simulink model "sldemo_variant_subsystems"  (Simulink 7.6)
settings: Solver=FixedStepDiscrete  StartTime=0.0  StopTime=10.0  RelTol=1e-3
PreLoadFcn:
  | VSS_NONLINEAR_CONTROLLER=Simulink.Variant('VSS_MODE==1')
  | VSS_SECOND_ORDER_CONTROLLER=Simulink.Variant('VSS_MODE==2')
  | 
  | VSS_MODE=1
Description:
  | Variant Subsystems
  | 
  | This demo illustrates Simulink(R) variant subsystems. Variant subsystems let
  | you provide multiple implementations to a subsystem where only one
  | implementation is active during simulation. You can programmatically swap out
  | the active implementation and replace it with one of the other implementations
  | without modifying the model.
settings Model: Creator=The MathWorks Inc.
settings OptimizationCC: InlineParams=on
settings RTWCC: ProcessScript=grt_make_rtw_hook

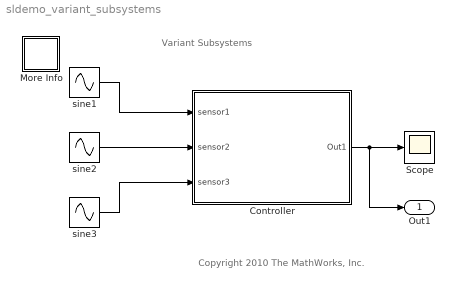
== system sldemo_variant_subsystems ==
  note: Copyright 2010 The MathWorks, Inc.
  note: Variant Subsystems
  Controller : Subsystem  Variant=on
  More Info : Subsystem
      settings: OpenFcn=showdemo(bdroot(gcb))
      mask Display: disp('?')
  Scope : Scope
  sine1 : Sin  Amplitude=.1  Frequency=pi/3  SampleTime=.01
  sine2 : Sin  Amplitude=2  SampleTime=.01
  sine3 : Sin  Amplitude=.3  Frequency=pi/6  SampleTime=.01
  Out1 : Outport
  wires:
  sine2/1 -> Controller/2(sensor2)
  sine1/1 -> Controller/1(sensor1)
  sine3/1 -> Controller/3(sensor3)
  Controller/1(Out1) -> Scope/1, Out1/1

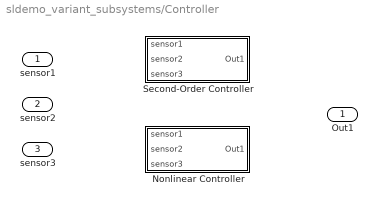
== system sldemo_variant_subsystems/Controller ==
  sensor1 : Inport
  sensor2 : Inport  Port=2
  sensor3 : Inport  Port=3
  Nonlinear Controller : Subsystem  VariantObject=VSS_NONLINEAR_CONTROLLER
  Second-Order Controller : Subsystem  VariantObject=VSS_SECOND_ORDER_CONTROLLER
  Out1 : Outport

== system sldemo_variant_subsystems/More Info ==
  note: This demo illustrates model reference variants. A Model block is used to
      | reference one Simulink model from another Simulink model. A Model block can
      | have different variants. A variant describes one of N possible modes a Model
      | block can operate in. Each variant of the Model block references a specific
      | model with model specific arguments. Only one variant is active for
      | simulation. You can switch the active variant of a Model block by changing the
      | values of variables in the base workspace or manually overriding variant
      | selection using the Model block dialog.
  note: Model Reference Variants

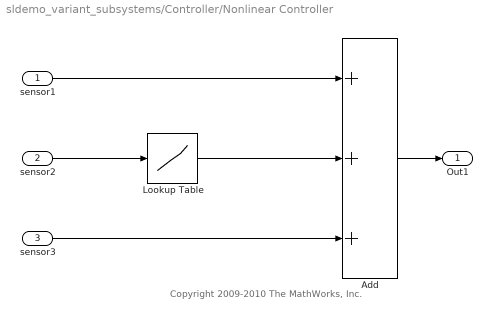
== system sldemo_variant_subsystems/Controller/Nonlinear Controller ==
  note: Copyright 2009-2010 The MathWorks, Inc.
  sensor1 : Inport
  sensor2 : Inport  Port=2
  sensor3 : Inport  Port=3
  Add : Sum  Inputs=+++  SampleTime=.01
  Lookup Table : Lookup  InputValues=[-5:5]  Table=tanh([-5:5])
  Out1 : Outport
  wires:
  sensor2/1 -> Lookup Table/1
  Lookup Table/1 -> Add/2
  sensor3/1 -> Add/3
  sensor1/1 -> Add/1
  Add/1 -> Out1/1

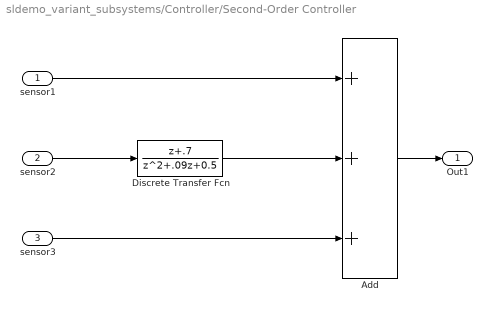
== system sldemo_variant_subsystems/Controller/Second-Order Controller ==
  sensor1 : Inport
  sensor2 : Inport  Port=2
  sensor3 : Inport  Port=3
  Add : Sum  Inputs=+++
  Discrete Transfer Fcn : DiscreteTransferFcn  Numerator=[1 .7]  Denominator=[1 .09 0.5]  SampleTime=.01
  Out1 : Outport
  wires:
  sensor2/1 -> Discrete Transfer Fcn/1
  Discrete Transfer Fcn/1 -> Add/2
  sensor3/1 -> Add/3
  sensor1/1 -> Add/1
  Add/1 -> Out1/1
